simulink model "CO2_Test"  (R2024a)
settings: Solver=FixedStepDiscrete  StartTime=0.0  StopTime=10.0  FixedStep=0.1  RelTol=1e-3
settings Model: Creator=Educação  LastModifiedBy=Gabriel

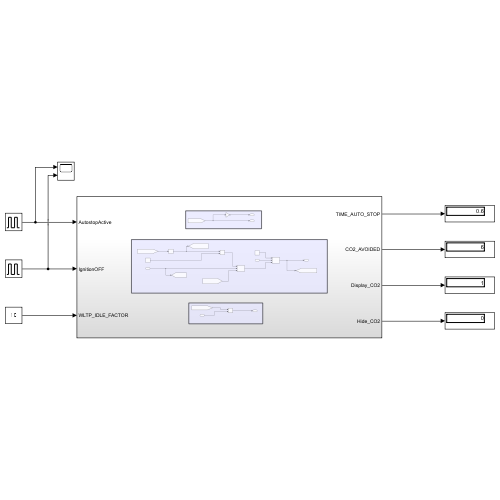
[thumbnail: Simulink's stored preview of the top-level diagram]
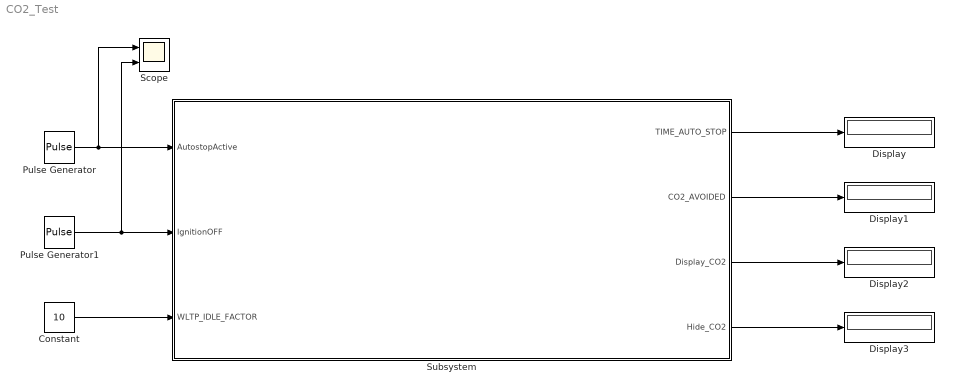
== system CO2_Test ==
  Constant : Constant  Value=10
  Display{,1..3} (4 alike) : Display
  Pulse Generator : DiscretePulseGenerator  PulseType=Time based  PulseWidth=50
  Pulse Generator1 : DiscretePulseGenerator  PulseType=Time based  Period=10  PulseWidth=5  PhaseDelay=8
  Scope : Scope  NumInputPorts=2
  Subsystem : Subsystem
  wires:
  Constant/1 -> Subsystem/3(WLTP_IDLE_FACTOR)
  Subsystem/1(TIME_AUTO_STOP) -> Display/1
  Subsystem/2(CO2_AVOIDED) -> Display1/1
  Pulse Generator/1 -> Scope/1, Subsystem/1(AutostopActive)
  Subsystem/3(Display_CO2) -> Display2/1
  Subsystem/4(Hide_CO2) -> Display3/1
  Pulse Generator1/1 -> Scope/2, Subsystem/2(IgnitionOFF)

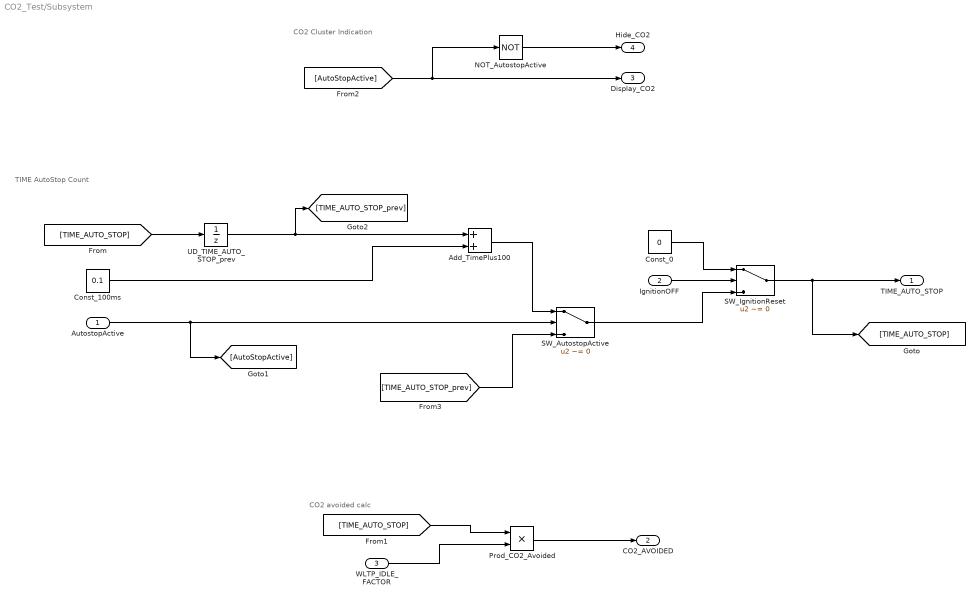
== system CO2_Test/Subsystem ==
  note: TIME AutoStop Count
  note: CO2 Cluster Indication
  note: CO2 avoided calc
  AutostopActive : Inport
  IgnitionOFF : Inport  Port=2
  WLTP_IDLE_FACTOR : Inport  Port=3
  Add_TimePlus100 : Sum
  Const_0 : Constant  Value=0
  Const_100ms : Constant  Value=0.1
  NOT_AutostopActive : Logic  Operator=NOT  IconShape=distinctive  AllPortsSameDT=off  OutDataTypeStr=boolean
  Prod_CO2_Avoided : Product
  SW_AutostopActive : Switch  Criteria=u2 ~= 0  SaturateOnIntegerOverflow=off  InputSameDT=off
  SW_IgnitionReset : Switch  Criteria=u2 ~= 0  SaturateOnIntegerOverflow=off  InputSameDT=off
  UD_TIME_AUTO_STOP_prev : UnitDelay  SampleTime=-1  HasFrameUpgradeWarning=on
  TIME_AUTO_STOP : Outport
  CO2_AVOIDED : Outport  Port=2
  Display_CO2 : Outport  Port=3
  Hide_CO2 : Outport  Port=4
  wires:
  UD_TIME_AUTO_STOP_prev/1 -> [TIME_AUTO_STOP_prev], Add_TimePlus100/1
  Const_100ms/1 -> Add_TimePlus100/2
  Add_TimePlus100/1 -> SW_AutostopActive/1
  AutostopActive/1 -> SW_AutostopActive/2, [AutoStopActive]
  Const_0/1 -> SW_IgnitionReset/1
  SW_AutostopActive/1 -> SW_IgnitionReset/3
  IgnitionOFF/1 -> SW_IgnitionReset/2
  SW_IgnitionReset/1 -> [TIME_AUTO_STOP], TIME_AUTO_STOP/1
  WLTP_IDLE_FACTOR/1 -> Prod_CO2_Avoided/2
  Prod_CO2_Avoided/1 -> CO2_AVOIDED/1
  NOT_AutostopActive/1 -> Hide_CO2/1
  [TIME_AUTO_STOP] -> UD_TIME_AUTO_STOP_prev/1
  [TIME_AUTO_STOP] -> Prod_CO2_Avoided/1
  [AutoStopActive] -> Display_CO2/1, NOT_AutostopActive/1
  [TIME_AUTO_STOP_prev] -> SW_AutostopActive/3
